simulink model "quadcopter"  (R2021b)
settings: Solver=VariableStepAuto  StartTime=0.0  StopTime=10.0  RelTol=1e-3
model workspace (MAT data in the model file):
  Ix = Simulink.Parameter
  Ix.DataType = 'auto'
  Ix.Complexity = 'real'
  Ix.Dimensions = [0 0]
  Iy = Simulink.Parameter
  Iy.DataType = 'auto'
  Iy.Complexity = 'real'
  Iy.Dimensions = [0 0]
  Iz = Simulink.Parameter
  Iz.DataType = 'auto'
  Iz.Complexity = 'real'
  Iz.Dimensions = [0 0]
  L = Simulink.Parameter
  L.DataType = 'auto'
  L.Complexity = 'real'
  L.Dimensions = [0 0]
  b = Simulink.Parameter
  b.DataType = 'auto'
  b.Complexity = 'real'
  b.Dimensions = [0 0]
  n11 = Simulink.Parameter
  n11.DataType = 'auto'
  n11.Complexity = 'real'
  n11.Dimensions = [0 0]
  n12 = Simulink.Parameter
  n12.DataType = 'auto'
  n12.Complexity = 'real'
  n12.Dimensions = [0 0]
  n13 = Simulink.Parameter
  n13.DataType = 'auto'
  n13.Complexity = 'real'
  n13.Dimensions = [0 0]
  n21 = Simulink.Parameter
  n21.DataType = 'auto'
  n21.Complexity = 'real'
  n21.Dimensions = [0 0]
  n22 = Simulink.Parameter
  n22.DataType = 'auto'
  n22.Complexity = 'real'
  n22.Dimensions = [0 0]
  n23 = Simulink.Parameter
  n23.DataType = 'auto'
  n23.Complexity = 'real'
  n23.Dimensions = [0 0]
  n31 = Simulink.Parameter
  n31.DataType = 'auto'
  n31.Complexity = 'real'
  n31.Dimensions = [0 0]
  n32 = Simulink.Parameter
  n32.DataType = 'auto'
  n32.Complexity = 'real'
  n32.Dimensions = [0 0]
  n33 = Simulink.Parameter
  n33.DataType = 'auto'
  n33.Complexity = 'real'
  n33.Dimensions = [0 0]
  v1 = Simulink.Parameter
  v1.DataType = 'auto'
  v1.Complexity = 'real'
  v1.Dimensions = [0 0]
  v2 = Simulink.Parameter
  v2.DataType = 'auto'
  v2.Complexity = 'real'
  v2.Dimensions = [0 0]
  v3 = Simulink.Parameter
  v3.DataType = 'auto'
  v3.Complexity = 'real'
  v3.Dimensions = [0 0]
  v4 = Simulink.Parameter
  v4.DataType = 'auto'
  v4.Complexity = 'real'
  v4.Dimensions = [0 0]
settings Model: Creator=collinlove  LastModifiedBy=collinlove

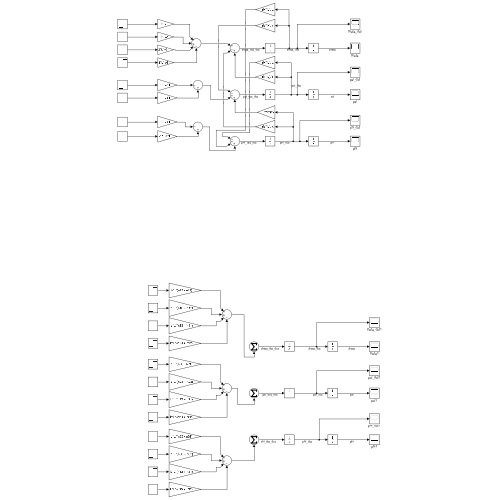
[thumbnail: Simulink's stored preview of the top-level diagram]
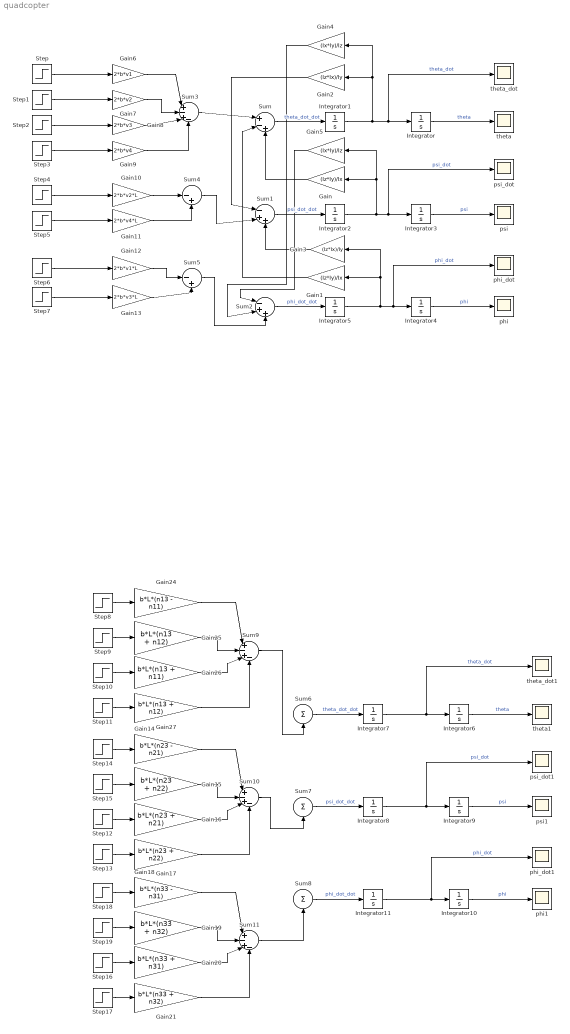
== system quadcopter ==
  Gain : Gain  Gain=(Iz*Iy)/Ix
  Gain1 : Gain  Gain=(Iz*Iy)/Ix
  Gain10 : Gain  Gain=2*b*v2*L
  Gain11 : Gain  Gain=2*b*v4*L
  Gain12 : Gain  Gain=2*b*v1*L
  Gain13 : Gain  Gain=2*b*v3*L
  Gain14 : Gain  Gain=b*L*(n23 - n21)
  Gain15 : Gain  Gain=b*L*(n23 + n22)
  Gain16 : Gain  Gain=b*L*(n23 + n21)
  Gain17 : Gain  Gain=b*L*(n23 + n22)
  Gain18 : Gain  Gain=b*L*(n33 - n31)
  Gain19 : Gain  Gain=b*L*(n33 + n32)
  Gain2 : Gain  Gain=(Iz*Ix)/Iy
  Gain20 : Gain  Gain=b*L*(n33 + n31)
  Gain21 : Gain  Gain=b*L*(n33 + n32)
  Gain24 : Gain  Gain=b*L*(n13 - n11)
  Gain25 : Gain  Gain=b*L*(n13 + n12)
  Gain26 : Gain  Gain=b*L*(n13 + n11)
  Gain27 : Gain  Gain=b*L*(n13 + n12)
  Gain3 : Gain  Gain=(Iz*Ix)/Iy
  Gain4 : Gain  Gain=(Ix*Iy)/Iz
  Gain5 : Gain  Gain=(Ix*Iy)/Iz
  Gain6 : Gain  Gain=2*b*v1
  Gain7 : Gain  Gain=2*b*v2
  Gain8 : Gain  Gain=2*b*v3
  Gain9 : Gain  Gain=2*b*v4
  Integrator{,1..11} (12 alike) : Integrator
  Step{,1..19} (20 alike) : Step  SampleTime=0
  Sum : Sum  Inputs=|+-+
  Sum1 : Sum  Inputs=|-++
  Sum{3,9..11} (4 alike) : Sum  Inputs=|+-+-
  Sum2 : Sum  Inputs=|-++
  Sum4 : Sum  Inputs=|-+
  Sum5 : Sum  Inputs=|-+
  Sum6 : Sum  Inputs=|+
  Sum7 : Sum  Inputs=|+
  Sum8 : Sum  Inputs=|+
  phi : Scope
  phi1 : Scope
  phi_dot : Scope
  phi_dot1 : Scope
  psi : Scope
  psi1 : Scope
  psi_dot : Scope
  psi_dot1 : Scope
  theta : Scope
  theta1 : Scope
  theta_dot : Scope
  theta_dot1 : Scope
  wires:
  Integrator1/1 -> Gain4/1, Gain2/1, Integrator/1, theta_dot/1  "theta_dot"
  Integrator/1 -> theta/1  "theta"
  Integrator2/1 -> Gain5/1, Gain/1, Integrator3/1, psi_dot/1  "psi_dot"
  Integrator5/1 -> Gain3/1, Gain1/1, Integrator4/1, phi_dot/1  "phi_dot"
  Integrator3/1 -> psi/1  "psi"
  Integrator4/1 -> phi/1  "phi"
  Sum/1 -> Integrator1/1  "theta_dot_dot"
  Gain/1 -> Sum/3
  Gain1/1 -> Sum/2
  Sum1/1 -> Integrator2/1  "psi_dot_dot"
  Gain2/1 -> Sum1/1
  Sum2/1 -> Integrator5/1  "phi_dot_dot"
  Gain3/1 -> Sum1/3
  Gain4/1 -> Sum2/2
  Gain5/1 -> Sum2/1
  Gain6/1 -> Sum3/1
  Gain7/1 -> Sum3/2
  Gain8/1 -> Sum3/3
  Gain9/1 -> Sum3/4
  Sum3/1 -> Sum/1
  Step/1 -> Gain6/1
  Step1/1 -> Gain7/1
  Step2/1 -> Gain8/1
  Step3/1 -> Gain9/1
  Gain10/1 -> Sum4/1
  Gain11/1 -> Sum4/2
  Sum4/1 -> Sum1/2
  Step4/1 -> Gain10/1
  Step5/1 -> Gain11/1
  Sum5/1 -> Sum2/3
  Gain12/1 -> Sum5/1
  Gain13/1 -> Sum5/2
  Step6/1 -> Gain12/1
  Step7/1 -> Gain13/1
  Gain25/1 -> Sum9/2
  Integrator7/1 -> Integrator6/1, theta_dot1/1  "theta_dot"
  Gain26/1 -> Sum9/3
  Gain27/1 -> Sum9/4
  Step9/1 -> Gain25/1
  Gain24/1 -> Sum9/1
  Integrator6/1 -> theta1/1  "theta"
  Integrator8/1 -> Integrator9/1, psi_dot1/1  "psi_dot"
  Integrator9/1 -> psi1/1  "psi"
  Integrator10/1 -> phi1/1  "phi"
  Step8/1 -> Gain24/1
  Integrator11/1 -> Integrator10/1, phi_dot1/1  "phi_dot"
  Sum8/1 -> Integrator11/1  "phi_dot_dot"
  Sum6/1 -> Integrator7/1  "theta_dot_dot"
  Step10/1 -> Gain26/1
  Step11/1 -> Gain27/1
  Sum7/1 -> Integrator8/1  "psi_dot_dot"
  Sum9/1 -> Sum6/1
  Step15/1 -> Gain15/1
  Step13/1 -> Gain17/1
  Step12/1 -> Gain16/1
  Gain14/1 -> Sum10/1
  Step14/1 -> Gain14/1
  Gain15/1 -> Sum10/2
  Gain17/1 -> Sum10/4
  Gain16/1 -> Sum10/3
  Sum10/1 -> Sum7/1
  Gain21/1 -> Sum11/4
  Gain19/1 -> Sum11/2
  Step19/1 -> Gain19/1
  Gain20/1 -> Sum11/3
  Gain18/1 -> Sum11/1
  Step18/1 -> Gain18/1
  Step16/1 -> Gain20/1
  Step17/1 -> Gain21/1
  Sum11/1 -> Sum8/1
